simulink model "Function2_2018a"  (R2018a)
settings: Solver=FixedStepDiscrete  StartTime=0.0  StopTime=0.1  FixedStep=0.1  RelTol=1e-3  EnableMultiTasking=on
settings Model: Creator=bzhan  LastModifiedBy=bzhan
settings SolverCC: AutoInsertRateTranBlk=on
settings DataIOCC: LimitDataPoints=on  ReturnWorkspaceOutputs=on
settings OptimizationCC: LifeSpan=inf
settings DebuggingCC: AllowSymbolicDim=off  SFUnexpectedBacktrackingDiag=warning  SFNoUnconditionalDefaultTransitionDiag=warning  SFExecutionAtInitializationDiag=none
settings CodeAppCC: StateflowObjectComments=on
settings GRTTargetCC: TargetLangStandard=C89/C90 (ANSI)
settings ConfigComp: CovMetricSettings=dw  CovHtmlReporting=on  CovSaveCumulativeToWorkspaceVar=on  CovSaveSingleToWorkspaceVar=on  CovShowResultsExplorer=off  CovExternalEMLEnable=off  CovSFcnEnable=off

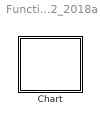
== system Function2_2018a ==
  Chart : Stateflow chart  TreatAsAtomicUnit=on

== stateflow chart Function2_2018a/Chart ==
  state A
    en: f("en_A")
  state B
    en: f("en_B")
  (default) -> A
  A -> (junction 29) : {[a,b]=compute2(3,4);}
  (junction 29) -> B : [a==10 && b==12]
  data: x function_input; w function_output double; y function_input; z function_output double; s function_input; a local; b local
  function [w,z] = compute2(x,y):
    | function [w,z] = compute2(x,y)
    |   x = x + 1;
    |   y = y - 1;
    |   w = x + 2 * y;
    |   z = x * y;
  function f(s):
    | function f(s)
    |   fprintf(s+"\n");
